simulink model "DemonstratorSimscape"  (R2020b)
settings: Solver=ode113  StartTime=0.0  StopTime=t_stop*0+20  FixedStep=1e-4
values from neighbouring files (symbols this model uses):
  brkD = 0    [main.m]
  brkI = 1e4    (= 10000)    [main.m]
  brkP = 1e5    (= 100000)    [main.m]
  d_drm = 0.5*d_drum    [main.m]
  d_shm = 0.4*d_sheave    [main.m]
  DeltaCable0 = 0    [main.m]
  Droop_scaling = 0    [main.m]
  eta_sh = 0.015    [main.m]
  filt_NUM = ones(1,200)*0.005    [main.m]
  g = 9.80665    [main.m]
  Iw = 0.5*(W.i + M.in*GB.r^2)    [main.m]
  Kp_mul = 0.3    [main.m]
  Lc0 = abs((T.ph-L.height-P.d-L.z0)*0.001)    [main.m]
  Ls1 = ((T.ph-0.5*W.pd)/1000)    [main.m]
  Ls2 = ((0.5*(T.s2+P.d)-2*P.d)/1000)    [main.m]
  M = 50e3    (= 50000)    [calcGrav.m]
  phi0_drm = -90    [main.m]
  phi0_shm = -90    [main.m]
  r_sheave = P.d*0.5    [main.m]
  s = tf('s')    [calcGrav.m]
  tau_brk = 0.001    [main.m]
  tau_em = 60e-3    (= 0.06)    [calcGrav.m]    (also in main.m)
  tau_m = tau_w/GB.r    [main.m]
  Tmax = 400e3    (= 400000)    [main.m]
  Tn_mul = 10    [main.m]
  x_drm = 0.7*r_drum    [main.m]
  x_shm = 0.7*r_sheave    [main.m]
  z0 = 0    [calcGrav.m]    (also in main.m = L.z0-P.d*0.5-P.d-P.d-L.height-T.h1-T.h2-32)
undefined symbols (not defined in the file or in its folder): C, CA, Controller_sampleTime, DiscIntNeverNeededParam, GB, L, P, Part, T, VFD_acceleration_model_factor, VFD_Adapt_factor_lower_p1458, VFD_Adapt_factor_upper_p1459, VFD_Curr_limit_var_p0641, VFD_Current_limit_p0640, VFD_Id_setp_total_r1624, VFD_Iq, VFD_Kp_n_basic_p1460, VFD_M, VFD_M_accel_T_smooth_p1517, VFD_M_lim_var_fixS_src_p1551, VFD_M_max_lower_p1521, VFD_M_max_lower_scal_p1525, VFD_M_max_up_mot_scal_p1524, VFD_M_max_upper_p1520, VFD_n_act_T_smooth_p1442, VFD_n_ctr_Kp_n_up_scal_p1461, VFD_n_ctr_Tn_n_up_sca_p1463, VFD_n_ctrl_adapt_Kp_lower_p1456, VFD_n_ctrl_adapt_Kp_upper_p1457, VFD_n_ctrl_Adpt_sig_Kp_p1455, VFD_n_ctrl_Kp_scal_p1466, VFD_n_ctrl_n_lower_p1464, VFD_n_ctrl_n_upper_p1465, VFD_n_ctrl_Tn_n_lower_p1462, VFD_n_limit_neg_p1086, VFD_n_limit_pos_p1083, VFD_n_limit_setp_p1063, VFD_n_max_p1082, VFD_n_set_filt_1_T_p1416, VFD_P_max_gen_p1531, VFD_P_max_mot_p1530, VFD_PU_I_outp_max_r0289, VFD_RFG_ramp_down_time_p1121, VFD_RFG_ramp_up_time_p1120, VFD_RFG_t_RD_scal_p1139, VFD_RFG_t_RU_scal_p1138, VSD, W, X, Y, Z
libraries: sm_lib x248, nesl_utility x128, simulink x49, pid_lib x4, cstblocks x2, simulink_extras x2
(part 4 of 10)

== system DemonstratorSimscape/Transmission System/Anchor and Load/CableFlex_Right ==
  disp [m] : Inport
  Inertia1 : sm_lib/Body Elements/Inertia  InertiaType=PointMass  Mass=0.00000001  MassUnits=kg  CenterOfMass=[0 0 0]  CenterOfMassUnits=m  MomentsOfInertia=[1 1 1]  MomentsOfInertiaUnits=kg*m^2  ProductsOfInertia=[0 0 0]  ProductsOfInertiaUnits=kg*m^2  GraphicType=None  MarkerShape=Inertia  MarkerSize=20  GraphicVisPropType=SimpleVisualProperties  GraphicDiffuseColor=[0.5 0.5 0.5]  GraphicSpecularColor=[0.5 0.5 0.5 1.0]  GraphicAmbientColor=[0.15 0.15 0.15 1.0]  GraphicEmissiveColor=[0.0 0.0 0.0 1.0]  GraphicShininess=75  GraphicOpacity=1.0
  Inertia2 : sm_lib/Body Elements/Inertia  InertiaType=PointMass  Mass=0.00000001  MassUnits=kg  CenterOfMass=[0 0 0]  CenterOfMassUnits=m  MomentsOfInertia=[1 1 1]  MomentsOfInertiaUnits=kg*m^2  ProductsOfInertia=[0 0 0]  ProductsOfInertiaUnits=kg*m^2  GraphicType=None  MarkerShape=Inertia  MarkerSize=20  GraphicVisPropType=SimpleVisualProperties  GraphicDiffuseColor=[0.5 0.5 0.5]  GraphicSpecularColor=[0.5 0.5 0.5 1.0]  GraphicAmbientColor=[0.15 0.15 0.15 1.0]  GraphicEmissiveColor=[0.0 0.0 0.0 1.0]  GraphicShininess=75  GraphicOpacity=1.0
  Prismatic Joint : sm_lib/Joints/Prismatic Joint  JointMode=Normal  SenseConstraintForce=off  SenseConstraintForceX=off  SenseConstraintForceY=off  SenseConstraintForceZ=off  SenseConstraintTorque=off  SenseConstraintTorqueX=off  SenseConstraintTorqueY=off  SenseConstraintTorqueZ=off  SenseTotalForce=off  SenseTotalForceX=off  SenseTotalForceY=off  SenseTotalForceZ=off  SenseTotalTorque=off  SenseTotalTorqueX=off  SenseTotalTorqueY=off  SenseTotalTorqueZ=off  CompositeWrenchDir=FollowerOnBase  CompositeWrenchFrame=BaseFrame  EquilibriumPosition=0  EquilibriumPositionUnits=m  SpringStiffness=0  SpringStiffnessUnits=N/m  DampingCoefficient=0  DampingCoefficientUnits=N/(m/s)  TorqueActuationMode=ComputedTorque  MotionActuationMode=InputMotion  SensePosition=off  SenseVelocity=off  SenseAcceleration=off  SenseTorqueForce=off  SenseLowerLimitTorqueForce=off  SenseUpperLimitTorqueForce=off  LowerLimitSpecify=off  LowerLimitBound=-1  LowerLimitBoundUnits=m  LowerLimitStiffness=1e6  LowerLimitStiffnessUnits=N/m  LowerLimitDamping=1e3  LowerLimitDampingUnits=N/(m/s)  LowerLimitTransitionRegionWidth=1e-4  LowerLimitTransitionRegionWidthUnits=m  UpperLimitSpecify=off  UpperLimitBound=1  UpperLimitBoundUnits=m  UpperLimitStiffness=1e6  UpperLimitStiffnessUnits=N/m  UpperLimitDamping=1e3  UpperLimitDampingUnits=N/(m/s)  UpperLimitTransitionRegionWidth=1e-4  UpperLimitTransitionRegionWidthUnits=m  PositionTargetSpecify=on  PositionTargetPriority=High  PositionTargetValue=DeltaCable0*0  PositionTargetValueUnits=mm  VelocityTargetSpecify=off  VelocityTargetPriority=High  VelocityTargetValue=0  VelocityTargetValueUnits=m/s
  Rigid Transform1 : sm_lib/Frames and Transforms/Rigid Transform  TranslationMethod=None  TranslationStandardOffset=0  TranslationLengthUnit=m  TranslationStandardAxis=+Z  TranslationCartesianOffset=[0 0 0]  TranslationROffset=0  TranslationROffsetUnits=m  TranslationZOffset=0  TranslationZOffsetUnits=m  TranslationThetaOffset=0  TranslationThetaOffsetUnits=deg  RotationMethod=StandardAxis  RotationAngleUnits=deg  RotationStandardAxis=+X  RotationAngle=-90  RotationArbitraryAxis=[0 0 1]  FollAlignAxisA=+X  BaseAlignAxisA=+Y  FollAlignAxisB=+Y  BaseAlignAxisB=+Z  RotationSequenceAxes=FollowerAxes  RotationSequence=XYX  RotationSequenceAngles=[0 0 0]  RotationSequenceAnglesUnits=deg  RotationMatrix=[1 0 0; 0 1 0; 0 0 1]
  Rigid Transform2 : sm_lib/Frames and Transforms/Rigid Transform  TranslationMethod=None  TranslationStandardOffset=0  TranslationLengthUnit=m  TranslationStandardAxis=+Z  TranslationCartesianOffset=[0 0 0]  TranslationROffset=0  TranslationROffsetUnits=m  TranslationZOffset=0  TranslationZOffsetUnits=m  TranslationThetaOffset=0  TranslationThetaOffsetUnits=deg  RotationMethod=StandardAxis  RotationAngleUnits=deg  RotationStandardAxis=+X  RotationAngle=90  RotationArbitraryAxis=[0 0 1]  FollAlignAxisA=+X  BaseAlignAxisA=+Y  FollAlignAxisB=+Y  BaseAlignAxisB=+Z  RotationSequenceAxes=FollowerAxes  RotationSequence=XYX  RotationSequenceAngles=[0 0 0]  RotationSequenceAnglesUnits=deg  RotationMatrix=[1 0 0; 0 1 0; 0 0 1]
  Simulink-PS Converter1 : nesl_utility/Simulink-PS Converter  PhysicalDomain=network_engine_domain  SubClassName=ps_input  LeftPortType=input  RightPortType=output  PseudoPeriodic=off  Frequencies=[]  NoiseDistribution=none  NoiseParameters=[]  Unit=m  AffineConversion=on  FilteringAndDerivatives=filter  SimscapeFilterOrder=2  InputFilterTimeConstant=0.001  UdotUserProvided=2
  F : PMIOPort  Side=Right
  B : PMIOPort  Port=2  Side=Left
  wires:
  disp [m]/1 -> Simulink-PS Converter1/1
  connections:
  B/RConn1 -- Rigid Transform2/LConn1
  Simulink-PS Converter1/RConn1 -- Prismatic Joint/LConn2
  Inertia2/RConn1 -- Prismatic Joint/LConn1 -- Rigid Transform1/LConn1
  Inertia1/RConn1 -- Prismatic Joint/RConn1 -- Rigid Transform2/RConn1
  F/RConn1 -- Rigid Transform1/RConn1

== system DemonstratorSimscape/Transmission System/Anchor and Load/CableRigid_Left ==
  F : PMIOPort  Side=Right
  B : PMIOPort  Port=2  Side=Left
  connections:
  B/RConn1 -- F/RConn1

== system DemonstratorSimscape/Transmission System/Anchor and Load/CableRigid_Right ==
  F : PMIOPort  Side=Right
  B : PMIOPort  Port=2  Side=Left
  connections:
  B/RConn1 -- F/RConn1

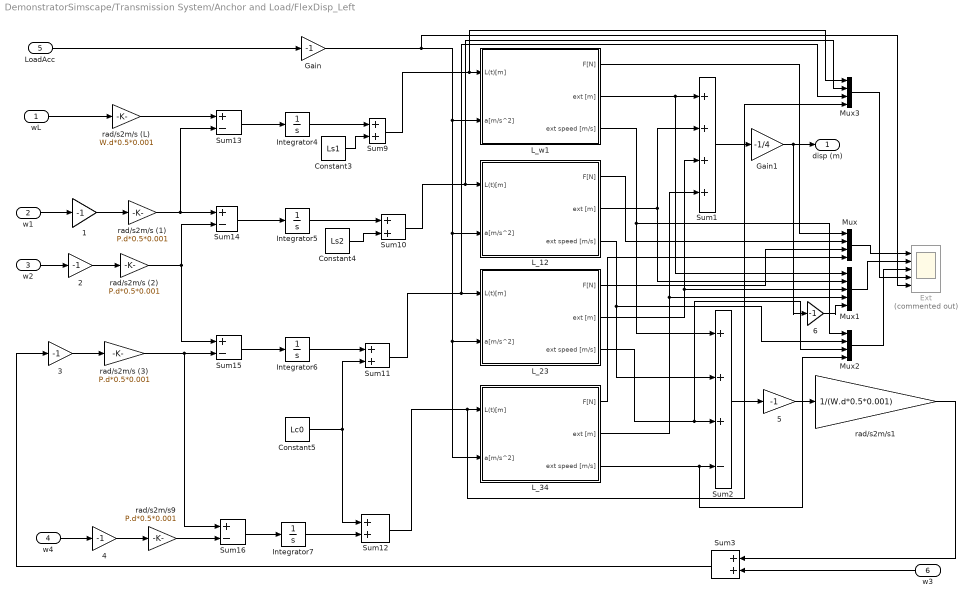
== system DemonstratorSimscape/Transmission System/Anchor and Load/FlexDisp_Left ==
  wL : Inport
  w1 : Inport  Port=2
  w2 : Inport  Port=3
  w4 : Inport  Port=4
  LoadAcc : Inport  Port=5
  w3 : Inport  Port=6
  {1..6} (6 alike) : Gain  Gain=-1
  Constant3 : Constant  Value=Ls1
  Constant4 : Constant  Value=Ls2
  Constant5 : Constant  Value=Lc0
  Ext : Scope  Commented=on  NumInputPorts=5
  Gain : Gain  Gain=-1
  Gain1 : Gain  Gain=-1/4
  Integrator{4..7} (4 alike) : Integrator
  L_12 : Subsystem
      settings: MinAlgLoopOccurrences=on
  L_23 : Subsystem
      settings: MinAlgLoopOccurrences=on
  L_34 : Subsystem
      settings: MinAlgLoopOccurrences=on
  L_w1 : Subsystem
      settings: MinAlgLoopOccurrences=on
  Mux : Mux
  Mux1 : Mux  Inputs=5
  Mux2 : Mux
  Mux3 : Mux
  Sum1 : Sum  Inputs=++++
  Sum{3,9..12} (5 alike) : Sum
  Sum{13..16} (4 alike) : Sum  Inputs=+-
  Sum2 : Sum  Inputs=+++-
  rad/s2m/s (1) : Gain  Gain=P.d*0.5*0.001
  rad/s2m/s (2) : Gain  Gain=P.d*0.5*0.001
  rad/s2m/s (3) : Gain  Gain=P.d*0.5*0.001
  rad/s2m/s (L) : Gain  Gain=W.d*0.5*0.001
  rad/s2m/s1 : Gain  Gain=1/(W.d*0.5*0.001)
  rad/s2m/s9 : Gain  Gain=P.d*0.5*0.001
  disp (m) : Outport
  wires:
  wL/1 -> rad/s2m/s (L)/1
  Integrator4/1 -> Sum9/1
  Sum15/1 -> Integrator6/1
  Sum9/1 -> Mux3/1, L_w1/1(L(t)[m])
  rad/s2m/s (1)/1 -> Sum14/1, Sum13/2
  LoadAcc/1 -> Gain/1
  Constant3/1 -> Sum9/2
  Sum12/1 -> Mux3/4, L_34/1(L(t)[m])
  Sum10/1 -> Mux3/2, L_12/1(L(t)[m])
  Integrator5/1 -> Sum10/1
  3/1 -> rad/s2m/s (3)/1
  2/1 -> rad/s2m/s (2)/1
  Sum13/1 -> Integrator4/1
  Constant5/1 -> Sum11/2, Sum12/1
  rad/s2m/s9/1 -> Sum16/2
  rad/s2m/s (L)/1 -> Sum13/1
  Integrator6/1 -> Sum11/1
  rad/s2m/s (3)/1 -> Sum15/2, Sum16/1
  w1/1 -> 1/1
  rad/s2m/s (2)/1 -> Sum14/2, Sum15/1
  4/1 -> rad/s2m/s9/1
  Constant4/1 -> Sum10/2
  Sum16/1 -> Integrator7/1
  w4/1 -> 4/1
  Sum14/1 -> Integrator5/1
  L_w1/2(ext [m]) -> Mux1/1, Sum1/1
  Sum11/1 -> Mux3/3, L_23/1(L(t)[m])
  1/1 -> rad/s2m/s (1)/1
  w2/1 -> 2/1
  Integrator7/1 -> Sum12/2
  Sum1/1 -> Gain1/1
  L_12/2(ext [m]) -> Sum1/2, Mux1/2
  L_23/2(ext [m]) -> Mux1/3, Sum1/3
  L_34/2(ext [m]) -> Mux1/4, Sum1/4
  Sum2/1 -> 5/1
  L_34/3(ext speed [m/s]) -> Mux2/4, Sum2/4
  L_23/3(ext speed [m/s]) -> Mux2/3, Sum2/3
  L_12/3(ext speed [m/s]) -> Mux2/2, Sum2/2
  L_w1/3(ext speed [m/s]) -> Mux2/1, Sum2/1
  5/1 -> rad/s2m/s1/1
  rad/s2m/s1/1 -> Sum3/1
  Sum3/1 -> 3/1
  Gain1/1 -> 6/1, disp (m)/1
  Gain/1 -> Ext/5, L_23/2(a[m/s^2]), L_34/2(a[m/s^2]), L_12/2(a[m/s^2]), L_w1/2(a[m/s^2])
  w3/1 -> Sum3/2
  Mux/1 -> Ext/1
  Mux1/1 -> Ext/2
  Mux2/1 -> Ext/3
  L_w1/1(F[N]) -> Mux/1
  L_12/1(F[N]) -> Mux/2
  L_23/1(F[N]) -> Mux/3
  L_34/1(F[N]) -> Mux/4
  6/1 -> Mux1/5
  Mux3/1 -> Ext/4

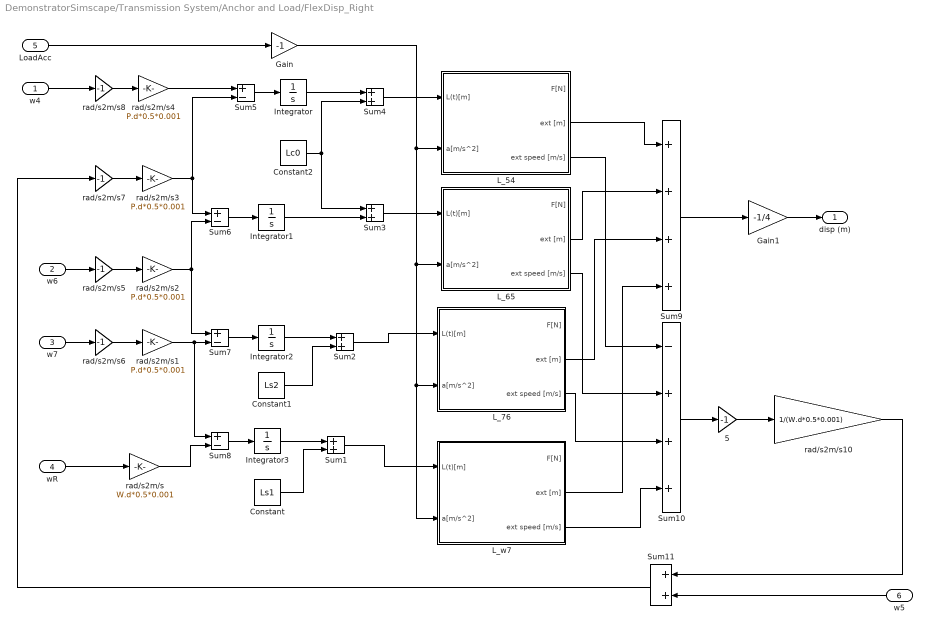
== system DemonstratorSimscape/Transmission System/Anchor and Load/FlexDisp_Right ==
  w4 : Inport
  w6 : Inport  Port=2
  w7 : Inport  Port=3
  wR : Inport  Port=4
  LoadAcc : Inport  Port=5
  w5 : Inport  Port=6
  5 : Gain  Gain=-1
  Constant : Constant  Value=Ls1
  Constant1 : Constant  Value=Ls2
  Constant2 : Constant  Value=Lc0
  Gain : Gain  Gain=-1
  Gain1 : Gain  Gain=-1/4
  Integrator{,1..3} (4 alike) : Integrator
  L_54 : Subsystem
      settings: MinAlgLoopOccurrences=on
  L_65 : Subsystem
      settings: MinAlgLoopOccurrences=on
  L_76 : Subsystem
      settings: MinAlgLoopOccurrences=on
  L_w7 : Subsystem
      settings: MinAlgLoopOccurrences=on
  Sum{1..4,11} (5 alike) : Sum
  Sum10 : Sum  Inputs=-+++
  Sum{5..8} (4 alike) : Sum  Inputs=+-
  Sum9 : Sum  Inputs=++++
  rad/s2m/s : Gain  Gain=W.d*0.5*0.001
  rad/s2m/s{1..4} (4 alike) : Gain  Gain=P.d*0.5*0.001
  rad/s2m/s10 : Gain  Gain=1/(W.d*0.5*0.001)
  rad/s2m/s{5..8} (4 alike) : Gain  Gain=-1
  disp (m) : Outport
  wires:
  Sum3/1 -> L_65/1(L(t)[m])
  w6/1 -> rad/s2m/s5/1
  LoadAcc/1 -> Gain/1
  Sum7/1 -> Integrator2/1
  Integrator/1 -> Sum4/1
  Sum4/1 -> L_54/1(L(t)[m])
  rad/s2m/s7/1 -> rad/s2m/s3/1
  rad/s2m/s3/1 -> Sum6/1, Sum5/2
  rad/s2m/s8/1 -> rad/s2m/s4/1
  w4/1 -> rad/s2m/s8/1
  rad/s2m/s6/1 -> rad/s2m/s1/1
  Constant2/1 -> Sum3/1, Sum4/2
  Sum8/1 -> Integrator3/1
  Sum2/1 -> L_76/1(L(t)[m])
  rad/s2m/s/1 -> Sum8/2
  Sum6/1 -> Integrator1/1
  Constant/1 -> Sum1/2
  rad/s2m/s5/1 -> rad/s2m/s2/1
  Sum5/1 -> Integrator/1
  Integrator2/1 -> Sum2/1
  rad/s2m/s2/1 -> Sum6/2, Sum7/1
  Constant1/1 -> Sum2/2
  Integrator1/1 -> Sum3/2
  Sum1/1 -> L_w7/1(L(t)[m])
  rad/s2m/s1/1 -> Sum7/2, Sum8/1
  w7/1 -> rad/s2m/s6/1
  Integrator3/1 -> Sum1/1
  rad/s2m/s4/1 -> Sum5/1
  wR/1 -> rad/s2m/s/1
  Gain/1 -> L_65/2(a[m/s^2]), L_76/2(a[m/s^2]), L_w7/2(a[m/s^2]), L_54/2(a[m/s^2])
  Sum9/1 -> Gain1/1
  L_54/2(ext [m]) -> Sum9/1
  L_65/2(ext [m]) -> Sum9/2
  L_76/2(ext [m]) -> Sum9/3
  L_w7/2(ext [m]) -> Sum9/4
  L_54/3(ext speed [m/s]) -> Sum10/1
  L_65/3(ext speed [m/s]) -> Sum10/2
  L_76/3(ext speed [m/s]) -> Sum10/3
  L_w7/3(ext speed [m/s]) -> Sum10/4
  rad/s2m/s10/1 -> Sum11/1
  Sum10/1 -> 5/1
  5/1 -> rad/s2m/s10/1
  Sum11/1 -> rad/s2m/s7/1
  w5/1 -> Sum11/2
  Gain1/1 -> disp (m)/1

== system DemonstratorSimscape/Transmission System/Anchor and Load/Load ==
  CableMass (kg) : Inport
  DOUBLE : Subsystem  Commented=on
  Load Sensors : Subsystem
  Pulley2 Rotation : sm_lib/Frames and Transforms/Rigid Transform  TranslationMethod=None  TranslationStandardOffset=0  TranslationLengthUnit=in  TranslationStandardAxis=+Z  TranslationCartesianOffset=[0 0 0]  TranslationROffset=0  TranslationROffsetUnits=m  TranslationZOffset=0  TranslationZOffsetUnits=m  TranslationThetaOffset=0  TranslationThetaOffsetUnits=deg  RotationMethod=StandardAxis  RotationAngleUnits=deg  RotationStandardAxis=+X  RotationAngle=-90  RotationArbitraryAxis=[0 0 1]  FollAlignAxisA=+Y  BaseAlignAxisA=+Z  FollAlignAxisB=+X  BaseAlignAxisB=+X  RotationSequenceAxes=FollowerAxes  RotationSequence=XYX  RotationSequenceAngles=[0 0 0]  RotationSequenceAnglesUnits=deg  RotationMatrix=[1 0 0; 0 1 0; 0 0 1]
  SINGLE : Subsystem
  F_Left : PMIOPort  Side=Left
  Centre : PMIOPort  Port=2  Side=Right
  F_Right : PMIOPort  Port=3  Side=Left
  LoadAcc (m/s^2) : Outport
  LoadPos (mm) : Outport  Port=2
  LoadVel (m/s) : Outport  Port=3
  wires:
  Load Sensors/2(LoadPos (mm)) -> LoadPos (mm)/1
  CableMass (kg)/1 -> DOUBLE/1(cable mass), SINGLE/1(cable mass)
  Load Sensors/1(LoadAcc (m/s^2)) -> LoadAcc (m/s^2)/1
  Load Sensors/3(LoadVel (m/s)) -> LoadVel (m/s)/1
  connections:
  DOUBLE/RConn2 -- F_Right/RConn1 -- SINGLE/RConn2
  SINGLE/LConn2 -- Load Sensors/RConn1 -- DOUBLE/LConn2
  SINGLE/LConn1 -- DOUBLE/LConn1 -- Pulley2 Rotation/RConn1
  DOUBLE/RConn1 -- SINGLE/RConn1 -- F_Left/RConn1
  Pulley2 Rotation/LConn1 -- Centre/RConn1

== system DemonstratorSimscape/Transmission System/Anchor and Load/Sheave_03 ==
  Bending loss : Subsystem  Commented=on
  Gain : Gain  Gain=-1
  Nm : nesl_utility/Simulink-PS Converter  PhysicalDomain=network_engine_domain  SubClassName=ps_input  LeftPortType=input  RightPortType=output  PseudoPeriodic=off  Frequencies=[]  NoiseDistribution=none  NoiseParameters=[]  Unit=1  AffineConversion=off  FilteringAndDerivatives=filter  SimscapeFilterOrder=2  InputFilterTimeConstant=tau_bending  UdotUserProvided=0
  PS>Sim1 : Subsystem
  Pulley 3 : sm_lib/Belts and Cables/Pulley  PitchRadius=P.d*0.5  PitchRadiusUnits=mm  InitialWrapAngleLowerBound=0.0  InitialWrapAngleLowerBoundUnits=deg  SenseWrapAngle=off  SensePulleyAngleA=off  SensePulleyAngleB=off  SenseFleetAngleA=off  SenseFleetAngleB=off
      settings: SourceProductBaseCode=MS
  Revolute Pulley3 : sm_lib/Joints/Revolute Joint  JointMode=Normal  SenseConstraintForce=on  SenseConstraintForceX=off  SenseConstraintForceY=off  SenseConstraintForceZ=off  SenseConstraintTorque=on  SenseConstraintTorqueX=off  SenseConstraintTorqueY=off  SenseConstraintTorqueZ=off  SenseTotalForce=on  SenseTotalForceX=off  SenseTotalForceY=off  SenseTotalForceZ=off  SenseTotalTorque=on  SenseTotalTorqueX=off  SenseTotalTorqueY=off  SenseTotalTorqueZ=off  CompositeWrenchDir=FollowerOnBase  CompositeWrenchFrame=BaseFrame  EquilibriumPosition=0  EquilibriumPositionUnits=deg  SpringStiffness=0  SpringStiffnessUnits=N*m/deg  DampingCoefficient=b_pulley  DampingCoefficientUnits=N*m/(deg/s)  TorqueActuationMode=InputTorque  MotionActuationMode=ComputedMotion  SensePosition=on  SenseVelocity=on  SenseAcceleration=on  SenseTorqueForce=on  SenseLowerLimitTorqueForce=off  SenseUpperLimitTorqueForce=off  LowerLimitSpecify=off  LowerLimitBound=-90  LowerLimitBoundUnits=deg  LowerLimitStiffness=1e4  LowerLimitStiffnessUnits=N*m/deg  LowerLimitDamping=10  LowerLimitDampingUnits=N*m/(deg/s)  LowerLimitTransitionRegionWidth=0.1  LowerLimitTransitionRegionWidthUnits=deg  UpperLimitSpecify=off  UpperLimitBound=90  UpperLimitBoundUnits=deg  UpperLimitStiffness=1e4  UpperLimitStiffnessUnits=N*m/deg  UpperLimitDamping=10  UpperLimitDampingUnits=N*m/(deg/s)  UpperLimitTransitionRegionWidth=0.1  UpperLimitTransitionRegionWidthUnits=deg  PositionTargetSpecify=off  PositionTargetPriority=High  PositionTargetValue=0  PositionTargetValueUnits=deg  VelocityTargetSpecify=off  VelocityTargetPriority=High  VelocityTargetValue=0  VelocityTargetValueUnits=deg/s
  ScopePulley3 : Scope  Commented=on  NumInputPorts=8
  Sheave3 : Subsystem
      mask Display: image('sm_cable_drive_right_angle_pulleyA_IMAGE.png');
  w0 (rad/s) : nesl_utility/PS-Simulink Converter  PhysicalDomain=network_engine_domain  SubClassName=ps_output  LeftPortType=input  RightPortType=output  PseudoPeriodic=off  Frequencies=[]  Unit=rad/s  AffineConversion=on
  WireA : PMIOPort  Side=Left
  ConnS3 : PMIOPort  Port=2  Side=Right
  WireB : PMIOPort  Port=3  Side=Left
  w (rad/s) : Outport
  tag scope: S3=global, w3=global
  wires:
  PS>Sim1/1(Out1) -> ScopePulley3/1
  PS>Sim1/2(Out2) -> ScopePulley3/2
  PS>Sim1/7(Out7) -> ScopePulley3/7
  PS>Sim1/3(Out3) -> ScopePulley3/3
  PS>Sim1/5(Out5) -> ScopePulley3/5
  PS>Sim1/4(Out4) -> ScopePulley3/4
  PS>Sim1/6(Out6) -> ScopePulley3/6
  PS>Sim1/8(Out8) -> ScopePulley3/8
  w0 (rad/s)/1 -> Gain/1, w (rad/s)/1
  [S2] -> Bending loss/1(Sin (kN))
  Bending loss/1(dT (Nm)) -> Nm/1
  Bending loss/2(Sout (kN)) -> [S3]
  Gain/1 -> [w3], Bending loss/2(w (deg/s))
  connections:
  Sheave3/LConn1 -- Revolute Pulley3/RConn1
  Revolute Pulley3/RConn9 -- PS>Sim1/LConn8
  Sheave3/RConn1 -- Pulley 3/LConn1
  WireA/RConn1 -- Pulley 3/RConn1
  Revolute Pulley3/RConn8 -- PS>Sim1/LConn7
  w0 (rad/s)/LConn1 -- Revolute Pulley3/RConn3 -- PS>Sim1/LConn2
  Revolute Pulley3/RConn4 -- PS>Sim1/LConn3
  Revolute Pulley3/RConn7 -- PS>Sim1/LConn6
  Revolute Pulley3/RConn5 -- PS>Sim1/LConn4
  Revolute Pulley3/RConn2 -- PS>Sim1/LConn1
  Revolute Pulley3/LConn1 -- ConnS3/RConn1
  Revolute Pulley3/RConn6 -- PS>Sim1/LConn5
  WireB/RConn1 -- Pulley 3/RConn2
  Nm/RConn1 -- Revolute Pulley3/LConn2

== system DemonstratorSimscape/Transmission System/Anchor and Load/Sheave_05 ==
  Bending loss : Subsystem  Commented=on
  Gain : Gain  Gain=-1
  Nm : nesl_utility/Simulink-PS Converter  PhysicalDomain=network_engine_domain  SubClassName=ps_input  LeftPortType=input  RightPortType=output  PseudoPeriodic=off  Frequencies=[]  NoiseDistribution=none  NoiseParameters=[]  Unit=1  AffineConversion=off  FilteringAndDerivatives=filter  SimscapeFilterOrder=2  InputFilterTimeConstant=tau_bending  UdotUserProvided=0
  PS>Sim2 : Subsystem
  Pulley 5 : sm_lib/Belts and Cables/Pulley  PitchRadius=P.d*0.5  PitchRadiusUnits=mm  InitialWrapAngleLowerBound=0.0  InitialWrapAngleLowerBoundUnits=deg  SenseWrapAngle=off  SensePulleyAngleA=off  SensePulleyAngleB=off  SenseFleetAngleA=off  SenseFleetAngleB=off
      settings: SourceProductBaseCode=MS
  Revolute Pulley5 : sm_lib/Joints/Revolute Joint  JointMode=Normal  SenseConstraintForce=on  SenseConstraintForceX=off  SenseConstraintForceY=off  SenseConstraintForceZ=off  SenseConstraintTorque=on  SenseConstraintTorqueX=off  SenseConstraintTorqueY=off  SenseConstraintTorqueZ=off  SenseTotalForce=on  SenseTotalForceX=off  SenseTotalForceY=off  SenseTotalForceZ=off  SenseTotalTorque=on  SenseTotalTorqueX=off  SenseTotalTorqueY=off  SenseTotalTorqueZ=off  CompositeWrenchDir=FollowerOnBase  CompositeWrenchFrame=BaseFrame  EquilibriumPosition=0  EquilibriumPositionUnits=deg  SpringStiffness=0  SpringStiffnessUnits=N*m/deg  DampingCoefficient=b_pulley  DampingCoefficientUnits=N*m/(deg/s)  TorqueActuationMode=InputTorque  MotionActuationMode=ComputedMotion  SensePosition=on  SenseVelocity=on  SenseAcceleration=on  SenseTorqueForce=on  SenseLowerLimitTorqueForce=off  SenseUpperLimitTorqueForce=off  LowerLimitSpecify=off  LowerLimitBound=-90  LowerLimitBoundUnits=deg  LowerLimitStiffness=1e4  LowerLimitStiffnessUnits=N*m/deg  LowerLimitDamping=10  LowerLimitDampingUnits=N*m/(deg/s)  LowerLimitTransitionRegionWidth=0.1  LowerLimitTransitionRegionWidthUnits=deg  UpperLimitSpecify=off  UpperLimitBound=90  UpperLimitBoundUnits=deg  UpperLimitStiffness=1e4  UpperLimitStiffnessUnits=N*m/deg  UpperLimitDamping=10  UpperLimitDampingUnits=N*m/(deg/s)  UpperLimitTransitionRegionWidth=0.1  UpperLimitTransitionRegionWidthUnits=deg  PositionTargetSpecify=off  PositionTargetPriority=High  PositionTargetValue=0  PositionTargetValueUnits=deg  VelocityTargetSpecify=off  VelocityTargetPriority=High  VelocityTargetValue=0  VelocityTargetValueUnits=deg/s
  ScopePulley5 : Scope  Commented=on  NumInputPorts=8
  Sheave5 : Subsystem
      mask Display: image('sm_cable_drive_right_angle_pulleyA_IMAGE.png');
  w (rad/s)1 : nesl_utility/PS-Simulink Converter  PhysicalDomain=network_engine_domain  SubClassName=ps_output  LeftPortType=input  RightPortType=output  PseudoPeriodic=off  Frequencies=[]  Unit=rad/s  AffineConversion=on
  ConnS5 : PMIOPort  Side=Right
  WireA : PMIOPort  Port=2  Side=Left
  WireB : PMIOPort  Port=3  Side=Left
  w (rad/s) : Outport
  tag scope: S4=global, w5=global
  wires:
  PS>Sim2/6(Out6) -> ScopePulley5/6
  PS>Sim2/3(Out3) -> ScopePulley5/3
  PS>Sim2/4(Out4) -> ScopePulley5/4
  PS>Sim2/7(Out7) -> ScopePulley5/7
  PS>Sim2/1(Out1) -> ScopePulley5/1
  PS>Sim2/5(Out5) -> ScopePulley5/5
  PS>Sim2/2(Out2) -> ScopePulley5/2
  PS>Sim2/8(Out8) -> ScopePulley5/8
  w (rad/s)1/1 -> Gain/1, w (rad/s)/1
  [S5] -> Bending loss/1(Sin (kN))
  Bending loss/1(dT (Nm)) -> Nm/1
  Bending loss/2(Sout (kN)) -> [S4]
  Gain/1 -> [w5], Bending loss/2(w (deg/s))
  connections:
  w (rad/s)1/LConn1 -- Revolute Pulley5/RConn3 -- PS>Sim2/LConn2
  WireB/RConn1 -- Pulley 5/RConn2
  Revolute Pulley5/RConn4 -- PS>Sim2/LConn3
  Revolute Pulley5/RConn6 -- PS>Sim2/LConn5
  Revolute Pulley5/RConn9 -- PS>Sim2/LConn8
  Revolute Pulley5/RConn7 -- PS>Sim2/LConn6
  Revolute Pulley5/RConn5 -- PS>Sim2/LConn4
  Revolute Pulley5/RConn8 -- PS>Sim2/LConn7
  Revolute Pulley5/RConn2 -- PS>Sim2/LConn1
  Sheave5/RConn1 -- Pulley 5/LConn1
  Sheave5/LConn1 -- Revolute Pulley5/RConn1
  Revolute Pulley5/LConn1 -- ConnS5/RConn1
  Pulley 5/RConn1 -- WireA/RConn1
  Nm/RConn1 -- Revolute Pulley5/LConn2

== system DemonstratorSimscape/Transmission System/Anchor and Load/cable mass ==
  "LoadPos [mm] " : Inport
  Add : Sum  Inputs=+-
  CableMass : Scope  Commented=on  NumInputPorts=2
  Constant : Constant  Value=P.up-W.pd*0.5
  Constant4 : Constant  Value=P.up
  Constant5 : Constant  Value=L.height
  Constant6 : Constant  Value=P.d
  Demux : Demux  Outputs=2
  Gain{,4,7,9} (4 alike) : Gain  Gain=CA.mpl
  Gain1 : Gain  Gain=2
  Gain10 : Gain  Gain=0.5
  Gain11 : Gain  Gain=0.5
  Gain12 : Gain  Gain=0.5
  Gain{2,5..6,8} (4 alike) : Gain  Gain=1/1000
  Gain3 : Gain  Gain=4
  Mux : Mux  Inputs=2
  Sum : Sum  Inputs=-+
  Sum1 : Sum  Inputs=+--
  Sum2 : Sum
  Sum3 : Sum
  net cable mass [kg] : Outport  VectorParamsAs1DForOutWhenUnconnected=off
  payout  [m] : Outport  Port=2  VectorParamsAs1DForOutWhenUnconnected=off
  cable mass [kg] : Outport  Port=3  VectorParamsAs1DForOutWhenUnconnected=off
  tag scope: LoadCableMass=global, WinchCableMass=global
  wires:
  Sum1/1 -> Gain3/1
  Constant5/1 -> Sum3/1
  Gain3/1 -> Add/1, Mux/2, Sum2/2, Sum/2
  Gain1/1 -> Add/2, Mux/1, Sum2/1, Sum/1
  Constant6/1 -> Sum3/2
  Constant4/1 -> Sum1/1
  Constant/1 -> Gain1/1
  Sum3/1 -> Sum1/2
  Sum/1 -> Gain5/1
  Gain/1 -> net cable mass [kg]/1
  Gain5/1 -> payout  [m]/1, Gain/1
  "LoadPos [mm] "/1 -> Sum1/3
  Mux/1 -> Gain6/1
  Gain6/1 -> Gain7/1
  Gain7/1 -> Gain10/1
  Sum2/1 -> Gain2/1
  Gain2/1 -> Gain4/1
  Gain4/1 -> cable mass [kg]/1
  Add/1 -> Gain8/1
  Gain8/1 -> Gain9/1
  Gain9/1 -> Gain11/1
  Gain10/1 -> Demux/1, CableMass/1
  Gain11/1 -> CableMass/2
  Gain12/1 -> [LoadCableMass]
  Demux/1 -> [WinchCableMass]
  Demux/2 -> Gain12/1

== system DemonstratorSimscape/Transmission System/Roof Pulley Set/ENDS ==
  Belt-Cable End : sm_lib/Belts and Cables/Belt-Cable End
      settings: SourceProductBaseCode=MS
  Belt-Cable End1 : sm_lib/Belts and Cables/Belt-Cable End
      settings: SourceProductBaseCode=MS
  Brick Solid : sm_lib/Body Elements/Brick Solid  GraphicAmbientColor=[0.15 0.15 0.15 1.0]  BasedOnType=Density  BrickDimensions=0.2*[1 1 1]  BrickDimensionUnits=m  CenterOfMass=[0 0 0]  CenterOfMassUnits=m  GraphicDiffuseColor=0.2*[1 1 1]  Density=0  DensityUnits=kg/m^3  DoExposeReferenceFrame=on  GraphicEmissiveColor=[0.0 0.0 0.0 1.0]  ExportEntireGeometry=off  SerializedFrames=<Frames/>  MarkerShape=Sphere  MarkerSize=10  GraphicType=FromGeometry  InertiaType=CalculateFromGeometry  Mass=1  MassUnits=kg  MomentsOfInertia=[1 1 1]  MomentsOfInertiaUnits=kg*m^2  GraphicOpacity=1.0  ProductsOfInertia=[0 0 0]  ProductsOfInertiaUnits=kg*m^2  GraphicShininess=75  GraphicSpecularColor=[0.5 0.5 0.5 1.0]  GraphicVisPropType=SimpleVisualProperties
  Brick Solid1 : sm_lib/Body Elements/Brick Solid  GraphicAmbientColor=[0.15 0.15 0.15 1.0]  BasedOnType=Density  BrickDimensions=0.2*[1 1 1]  BrickDimensionUnits=m  CenterOfMass=[0 0 0]  CenterOfMassUnits=m  GraphicDiffuseColor=0.2*[1 1 1]  Density=0  DensityUnits=kg/m^3  DoExposeReferenceFrame=on  GraphicEmissiveColor=[0.0 0.0 0.0 1.0]  ExportEntireGeometry=off  SerializedFrames=<Frames/>  MarkerShape=Sphere  MarkerSize=10  GraphicType=FromGeometry  InertiaType=CalculateFromGeometry  Mass=1  MassUnits=kg  MomentsOfInertia=[1 1 1]  MomentsOfInertiaUnits=kg*m^2  GraphicOpacity=1.0  ProductsOfInertia=[0 0 0]  ProductsOfInertiaUnits=kg*m^2  GraphicShininess=75  GraphicSpecularColor=[0.5 0.5 0.5 1.0]  GraphicVisPropType=SimpleVisualProperties
  Demux : Demux  Outputs=3
  Demux1 : Demux  Outputs=3
  Ends Tension : Scope  Commented=on
  Mux : Mux
  PS-Simulink Converter : nesl_utility/PS-Simulink Converter  PhysicalDomain=network_engine_domain  SubClassName=ps_output  LeftPortType=input  RightPortType=output  PseudoPeriodic=off  Frequencies=[]  Unit=kN  AffineConversion=off
  PS-Simulink Converter1 : nesl_utility/PS-Simulink Converter  PhysicalDomain=network_engine_domain  SubClassName=ps_output  LeftPortType=input  RightPortType=output  PseudoPeriodic=off  Frequencies=[]  Unit=kN  AffineConversion=off
  Rigid Transform1 : sm_lib/Frames and Transforms/Rigid Transform  TranslationMethod=Cartesian  TranslationStandardOffset=0  TranslationLengthUnit=mm  TranslationStandardAxis=+Z  TranslationCartesianOffset="[-P.Bd*0.5  0 0]"  TranslationROffset=0  TranslationROffsetUnits=m  TranslationZOffset=0  TranslationZOffsetUnits=m  TranslationThetaOffset=0  TranslationThetaOffsetUnits=deg  RotationMethod=None  RotationAngleUnits=deg  RotationStandardAxis=+Z  RotationAngle=0.0  RotationArbitraryAxis=[0 0 1]  FollAlignAxisA=+X  BaseAlignAxisA=+Y  FollAlignAxisB=+Y  BaseAlignAxisB=+Z  RotationSequenceAxes=FollowerAxes  RotationSequence=XYX  RotationSequenceAngles=[0 0 0]  RotationSequenceAnglesUnits=deg  RotationMatrix=[1 0 0; 0 1 0; 0 0 1]
  Rigid Transform3 : sm_lib/Frames and Transforms/Rigid Transform  TranslationMethod=Cartesian  TranslationStandardOffset=0  TranslationLengthUnit=mm  TranslationStandardAxis=+Z  TranslationCartesianOffset="[P.Bd*0.5  0 0]"  TranslationROffset=0  TranslationROffsetUnits=m  TranslationZOffset=0  TranslationZOffsetUnits=m  TranslationThetaOffset=0  TranslationThetaOffsetUnits=deg  RotationMethod=None  RotationAngleUnits=deg  RotationStandardAxis=+Z  RotationAngle=0.0  RotationArbitraryAxis=[0 0 1]  FollAlignAxisA=+X  BaseAlignAxisA=+Y  FollAlignAxisB=+Y  BaseAlignAxisB=+Z  RotationSequenceAxes=FollowerAxes  RotationSequence=XYX  RotationSequenceAngles=[0 0 0]  RotationSequenceAnglesUnits=deg  RotationMatrix=[1 0 0; 0 1 0; 0 0 1]
  Weld Joint : sm_lib/Joints/Weld Joint  JointMode=Normal  SenseConstraintForce=on  SenseConstraintForceX=off  SenseConstraintForceY=off  SenseConstraintForceZ=off  SenseConstraintTorque=off  SenseConstraintTorqueX=off  SenseConstraintTorqueY=off  SenseConstraintTorqueZ=off  SenseTotalForce=off  SenseTotalForceX=off  SenseTotalForceY=off  SenseTotalForceZ=off  SenseTotalTorque=off  SenseTotalTorqueX=off  SenseTotalTorqueY=off  SenseTotalTorqueZ=off  CompositeWrenchDir=BaseOnFollower  CompositeWrenchFrame=FollowerFrame
  Weld Joint1 : sm_lib/Joints/Weld Joint  JointMode=Normal  SenseConstraintForce=on  SenseConstraintForceX=off  SenseConstraintForceY=off  SenseConstraintForceZ=off  SenseConstraintTorque=off  SenseConstraintTorqueX=off  SenseConstraintTorqueY=off  SenseConstraintTorqueZ=off  SenseTotalForce=off  SenseTotalForceX=off  SenseTotalForceY=off  SenseTotalForceZ=off  SenseTotalTorque=off  SenseTotalTorqueX=off  SenseTotalTorqueY=off  SenseTotalTorqueZ=off  CompositeWrenchDir=BaseOnFollower  CompositeWrenchFrame=FollowerFrame
  ConnCentre : PMIOPort  Side=Left
  ConnEndL : PMIOPort  Port=2  Side=Right
  ConnEndR : PMIOPort  Port=3  Side=Right
  wires:
  PS-Simulink Converter/1 -> Demux/1
  PS-Simulink Converter1/1 -> Demux1/1
  Demux1/2 -> Mux/2
  Mux/1 -> Ends Tension/1
  Demux/2 -> Mux/1
  [S3] -> Mux/3
  [S4] -> Mux/4
  connections:
  ConnEndL/RConn1 -- Belt-Cable End1/RConn1
  Rigid Transform3/LConn1 -- Rigid Transform1/LConn1 -- ConnCentre/RConn1
  Weld Joint/RConn1 -- Belt-Cable End/LConn1
  Rigid Transform1/RConn1 -- Brick Solid1/RConn1 -- Weld Joint1/LConn1
  ConnEndR/RConn1 -- Belt-Cable End/RConn1
  Rigid Transform3/RConn1 -- Brick Solid/RConn1 -- Weld Joint/LConn1
  Weld Joint1/RConn1 -- Belt-Cable End1/LConn1
  Weld Joint/RConn2 -- PS-Simulink Converter/LConn1
  PS-Simulink Converter1/LConn1 -- Weld Joint1/RConn2

== system DemonstratorSimscape/Transmission System/Roof Pulley Set/Sheave_01 ==
  " " : sm_lib/Frames and Transforms/Rigid Transform  TranslationMethod=Cartesian  TranslationStandardOffset=0  TranslationLengthUnit=mm  TranslationStandardAxis=+Z  TranslationCartesianOffset=[0 -P.d*.25 -P.h]  TranslationROffset=0  TranslationROffsetUnits=m  TranslationZOffset=0  TranslationZOffsetUnits=m  TranslationThetaOffset=0  TranslationThetaOffsetUnits=deg  RotationMethod=ArbitraryAxis  RotationAngleUnits=deg  RotationStandardAxis=+Z  RotationAngle=90  RotationArbitraryAxis=[1 0 0]  FollAlignAxisA=+X  BaseAlignAxisA=+Y  FollAlignAxisB=+Y  BaseAlignAxisB=+Z  RotationSequenceAxes=FollowerAxes  RotationSequence=XYX  RotationSequenceAngles=[0 0 0]  RotationSequenceAnglesUnits=deg  RotationMatrix=[1 0 0; 0 1 0; 0 0 1]
  " 4" : sm_lib/Frames and Transforms/Rigid Transform  TranslationMethod=Cartesian  TranslationStandardOffset=0  TranslationLengthUnit=mm  TranslationStandardAxis=+Z  TranslationCartesianOffset=[0 -P.d*.25 P.h]  TranslationROffset=0  TranslationROffsetUnits=m  TranslationZOffset=0  TranslationZOffsetUnits=m  TranslationThetaOffset=0  TranslationThetaOffsetUnits=deg  RotationMethod=ArbitraryAxis  RotationAngleUnits=deg  RotationStandardAxis=+Z  RotationAngle=90  RotationArbitraryAxis=[1 0 0]  FollAlignAxisA=+X  BaseAlignAxisA=+Y  FollAlignAxisB=+Y  BaseAlignAxisB=+Z  RotationSequenceAxes=FollowerAxes  RotationSequence=XYX  RotationSequenceAngles=[0 0 0]  RotationSequenceAnglesUnits=deg  RotationMatrix=[1 0 0; 0 1 0; 0 0 1]
  Bending loss : Subsystem  Commented=on
  Gain : Gain
  Nm : nesl_utility/Simulink-PS Converter  PhysicalDomain=network_engine_domain  SubClassName=ps_input  LeftPortType=input  RightPortType=output  PseudoPeriodic=off  Frequencies=[]  NoiseDistribution=none  NoiseParameters=[]  Unit=1  AffineConversion=off  FilteringAndDerivatives=filter  SimscapeFilterOrder=2  InputFilterTimeConstant=tau_bending  UdotUserProvided=0
  PS>Sim1 : Subsystem
  Pulley 1 : sm_lib/Belts and Cables/Pulley  PitchRadius=P.d*0.5  PitchRadiusUnits=mm  InitialWrapAngleLowerBound=0.0  InitialWrapAngleLowerBoundUnits=deg  SenseWrapAngle=off  SensePulleyAngleA=off  SensePulleyAngleB=off  SenseFleetAngleA=off  SenseFleetAngleB=off
      settings: SourceProductBaseCode=MS
  Revolute Pulley1 : sm_lib/Joints/Revolute Joint  JointMode=Normal  SenseConstraintForce=on  SenseConstraintForceX=off  SenseConstraintForceY=off  SenseConstraintForceZ=off  SenseConstraintTorque=on  SenseConstraintTorqueX=off  SenseConstraintTorqueY=off  SenseConstraintTorqueZ=off  SenseTotalForce=on  SenseTotalForceX=off  SenseTotalForceY=off  SenseTotalForceZ=off  SenseTotalTorque=on  SenseTotalTorqueX=off  SenseTotalTorqueY=off  SenseTotalTorqueZ=off  CompositeWrenchDir=FollowerOnBase  CompositeWrenchFrame=BaseFrame  EquilibriumPosition=0  EquilibriumPositionUnits=deg  SpringStiffness=0  SpringStiffnessUnits=N*m/deg  DampingCoefficient=b_pulley  DampingCoefficientUnits=N*m/(deg/s)  TorqueActuationMode=InputTorque  MotionActuationMode=ComputedMotion  SensePosition=on  SenseVelocity=on  SenseAcceleration=on  SenseTorqueForce=on  SenseLowerLimitTorqueForce=off  SenseUpperLimitTorqueForce=off  LowerLimitSpecify=off  LowerLimitBound=-90  LowerLimitBoundUnits=deg  LowerLimitStiffness=1e4  LowerLimitStiffnessUnits=N*m/deg  LowerLimitDamping=10  LowerLimitDampingUnits=N*m/(deg/s)  LowerLimitTransitionRegionWidth=0.1  LowerLimitTransitionRegionWidthUnits=deg  UpperLimitSpecify=off  UpperLimitBound=90  UpperLimitBoundUnits=deg  UpperLimitStiffness=1e4  UpperLimitStiffnessUnits=N*m/deg  UpperLimitDamping=10  UpperLimitDampingUnits=N*m/(deg/s)  UpperLimitTransitionRegionWidth=0.1  UpperLimitTransitionRegionWidthUnits=deg  PositionTargetSpecify=off  PositionTargetPriority=High  PositionTargetValue=0  PositionTargetValueUnits=deg  VelocityTargetSpecify=off  VelocityTargetPriority=High  VelocityTargetValue=0  VelocityTargetValueUnits=deg/s
  ScopePulley1 : Scope  Commented=on  NumInputPorts=8
  Sheave1 : Subsystem
      mask Display: image('sm_cable_drive_right_angle_pulleyA_IMAGE.png');
  left face : sm_lib/Body Elements/Brick Solid  GraphicAmbientColor=[0.15 0.15 0.15 1.0]  BasedOnType=Density  BrickDimensions=[P.d P.h P.d*.5]  BrickDimensionUnits=mm  CenterOfMass=[0 0 0]  CenterOfMassUnits=m  GraphicDiffuseColor=[0.6 0.6 0.0]  Density=0  DensityUnits=g/cm^3  DoExposeReferenceFrame=on  GraphicEmissiveColor=[0.0 0.0 0.0 1.0]  ExportEntireGeometry=off  SerializedFrames=<Frames/>  MarkerShape=Sphere  MarkerSize=10  GraphicType=FromGeometry  InertiaType=CalculateFromGeometry  Mass=1  MassUnits=kg  MomentsOfInertia=[1 1 1]  MomentsOfInertiaUnits=kg*m^2  GraphicOpacity=c.opac  ProductsOfInertia=[0 0 0]  ProductsOfInertiaUnits=kg*m^2  GraphicShininess=75  GraphicSpecularColor=[0.5 0.5 0.5 1.0]  GraphicVisPropType=SimpleVisualProperties
  right face : sm_lib/Body Elements/Brick Solid  GraphicAmbientColor=[0.15 0.15 0.15 1.0]  BasedOnType=Density  BrickDimensions=[P.d P.h P.d*.5]  BrickDimensionUnits=mm  CenterOfMass=[0 0 0]  CenterOfMassUnits=m  GraphicDiffuseColor=[0.6 0.6 0.0]  Density=0  DensityUnits=g/cm^3  DoExposeReferenceFrame=on  GraphicEmissiveColor=[0.0 0.0 0.0 1.0]  ExportEntireGeometry=off  SerializedFrames=<Frames/>  MarkerShape=Sphere  MarkerSize=10  GraphicType=FromGeometry  InertiaType=CalculateFromGeometry  Mass=1  MassUnits=kg  MomentsOfInertia=[1 1 1]  MomentsOfInertiaUnits=kg*m^2  GraphicOpacity=1.0  ProductsOfInertia=[0 0 0]  ProductsOfInertiaUnits=kg*m^2  GraphicShininess=75  GraphicSpecularColor=[0.5 0.5 0.5 1.0]  GraphicVisPropType=SimpleVisualProperties
  w (rad/s)1 : nesl_utility/PS-Simulink Converter  PhysicalDomain=network_engine_domain  SubClassName=ps_output  LeftPortType=input  RightPortType=output  PseudoPeriodic=off  Frequencies=[]  Unit=rad/s  AffineConversion=off
  WireA : PMIOPort  Side=Right
  Conn1 : PMIOPort  Port=2  Side=Left
  WireB : PMIOPort  Port=3  Side=Right
  w (rad/s) : Outport
  tag scope: S1=global, w1=global
  wires:
  w (rad/s)1/1 -> [w1], Gain/1, w (rad/s)/1
  PS>Sim1/5(Out5) -> ScopePulley1/5
  PS>Sim1/8(Out8) -> ScopePulley1/8
  PS>Sim1/2(Out2) -> ScopePulley1/2
  PS>Sim1/1(Out1) -> ScopePulley1/1
  PS>Sim1/3(Out3) -> ScopePulley1/3
  PS>Sim1/7(Out7) -> ScopePulley1/7
  PS>Sim1/4(Out4) -> ScopePulley1/4
  PS>Sim1/6(Out6) -> ScopePulley1/6
  Bending loss/1(dT (Nm)) -> Nm/1
  Bending loss/2(Sout (kN)) -> [S1]
  [S0] -> Bending loss/1(Sin (kN))
  Gain/1 -> Bending loss/2(w (deg/s))
  connections:
  Pulley 1/RConn1 -- WireA/RConn1
  Sheave1/RConn1 -- Pulley 1/LConn1
  Pulley 1/RConn2 -- WireB/RConn1
  PS>Sim1/LConn2 -- Revolute Pulley1/RConn3 -- w (rad/s)1/LConn1
  " 4"/LConn1 -- " "/LConn1 -- Conn1/RConn1 -- Revolute Pulley1/LConn1
  Revolute Pulley1/RConn6 -- PS>Sim1/LConn5
  Revolute Pulley1/RConn2 -- PS>Sim1/LConn1
  Sheave1/LConn1 -- Revolute Pulley1/RConn1
  " "/RConn1 -- right face/RConn1
  Revolute Pulley1/RConn4 -- PS>Sim1/LConn3
  Revolute Pulley1/RConn9 -- PS>Sim1/LConn8
  Revolute Pulley1/RConn8 -- PS>Sim1/LConn7
  Revolute Pulley1/RConn5 -- PS>Sim1/LConn4
  Revolute Pulley1/RConn7 -- PS>Sim1/LConn6
  " 4"/RConn1 -- left face/RConn1
  Nm/RConn1 -- Revolute Pulley1/LConn2

== system DemonstratorSimscape/Transmission System/Roof Pulley Set/Sheave_02 ==
  " " : sm_lib/Frames and Transforms/Rigid Transform  TranslationMethod=Cartesian  TranslationStandardOffset=0  TranslationLengthUnit=mm  TranslationStandardAxis=+Z  TranslationCartesianOffset=[0 -P.d*.25 -P.h]  TranslationROffset=0  TranslationROffsetUnits=m  TranslationZOffset=0  TranslationZOffsetUnits=m  TranslationThetaOffset=0  TranslationThetaOffsetUnits=deg  RotationMethod=ArbitraryAxis  RotationAngleUnits=deg  RotationStandardAxis=+Z  RotationAngle=90  RotationArbitraryAxis=[1 0 0]  FollAlignAxisA=+X  BaseAlignAxisA=+Y  FollAlignAxisB=+Y  BaseAlignAxisB=+Z  RotationSequenceAxes=FollowerAxes  RotationSequence=XYX  RotationSequenceAngles=[0 0 0]  RotationSequenceAnglesUnits=deg  RotationMatrix=[1 0 0; 0 1 0; 0 0 1]
  " 4" : sm_lib/Frames and Transforms/Rigid Transform  TranslationMethod=Cartesian  TranslationStandardOffset=0  TranslationLengthUnit=mm  TranslationStandardAxis=+Z  TranslationCartesianOffset=[0 -P.d*.25 P.h]  TranslationROffset=0  TranslationROffsetUnits=m  TranslationZOffset=0  TranslationZOffsetUnits=m  TranslationThetaOffset=0  TranslationThetaOffsetUnits=deg  RotationMethod=ArbitraryAxis  RotationAngleUnits=deg  RotationStandardAxis=+Z  RotationAngle=90  RotationArbitraryAxis=[1 0 0]  FollAlignAxisA=+X  BaseAlignAxisA=+Y  FollAlignAxisB=+Y  BaseAlignAxisB=+Z  RotationSequenceAxes=FollowerAxes  RotationSequence=XYX  RotationSequenceAngles=[0 0 0]  RotationSequenceAnglesUnits=deg  RotationMatrix=[1 0 0; 0 1 0; 0 0 1]
  Bending loss : Subsystem  Commented=on
  Constant : Constant  Value=g*1000
  Demux : Demux  Outputs=3
  Divide : Product  Inputs=*/
  Gain : Gain
  Gain1 : Gain  Gain=-2
  Nm : nesl_utility/Simulink-PS Converter  PhysicalDomain=network_engine_domain  SubClassName=ps_input  LeftPortType=input  RightPortType=output  PseudoPeriodic=off  Frequencies=[]  NoiseDistribution=none  NoiseParameters=[]  Unit=1  AffineConversion=off  FilteringAndDerivatives=filter  SimscapeFilterOrder=2  InputFilterTimeConstant=tau_bending  UdotUserProvided=0
  PS>Sim1 : Subsystem
  Pulley 2 : sm_lib/Belts and Cables/Pulley  PitchRadius=P.d*0.5  PitchRadiusUnits=mm  InitialWrapAngleLowerBound=0.0  InitialWrapAngleLowerBoundUnits=deg  SenseWrapAngle=off  SensePulleyAngleA=off  SensePulleyAngleB=off  SenseFleetAngleA=off  SenseFleetAngleB=off
      settings: SourceProductBaseCode=MS
  Revolute Pulley2 : sm_lib/Joints/Revolute Joint  JointMode=Normal  SenseConstraintForce=on  SenseConstraintForceX=off  SenseConstraintForceY=off  SenseConstraintForceZ=off  SenseConstraintTorque=on  SenseConstraintTorqueX=off  SenseConstraintTorqueY=off  SenseConstraintTorqueZ=off  SenseTotalForce=on  SenseTotalForceX=off  SenseTotalForceY=off  SenseTotalForceZ=off  SenseTotalTorque=on  SenseTotalTorqueX=off  SenseTotalTorqueY=off  SenseTotalTorqueZ=off  CompositeWrenchDir=FollowerOnBase  CompositeWrenchFrame=BaseFrame  EquilibriumPosition=0  EquilibriumPositionUnits=deg  SpringStiffness=0  SpringStiffnessUnits=N*m/deg  DampingCoefficient=b_pulley  DampingCoefficientUnits=N*m/(deg/s)  TorqueActuationMode=InputTorque  MotionActuationMode=ComputedMotion  SensePosition=on  SenseVelocity=on  SenseAcceleration=on  SenseTorqueForce=on  SenseLowerLimitTorqueForce=off  SenseUpperLimitTorqueForce=off  LowerLimitSpecify=off  LowerLimitBound=-90  LowerLimitBoundUnits=deg  LowerLimitStiffness=1e4  LowerLimitStiffnessUnits=N*m/deg  LowerLimitDamping=10  LowerLimitDampingUnits=N*m/(deg/s)  LowerLimitTransitionRegionWidth=0.1  LowerLimitTransitionRegionWidthUnits=deg  UpperLimitSpecify=off  UpperLimitBound=90  UpperLimitBoundUnits=deg  UpperLimitStiffness=1e4  UpperLimitStiffnessUnits=N*m/deg  UpperLimitDamping=10  UpperLimitDampingUnits=N*m/(deg/s)  UpperLimitTransitionRegionWidth=0.1  UpperLimitTransitionRegionWidthUnits=deg  PositionTargetSpecify=off  PositionTargetPriority=High  PositionTargetValue=0  PositionTargetValueUnits=deg  VelocityTargetSpecify=off  VelocityTargetPriority=High  VelocityTargetValue=0  VelocityTargetValueUnits=deg/s
  ScopePulley2 : Scope  Commented=on  NumInputPorts=8
  Sheave2 : Subsystem
      mask Display: image('sm_cable_drive_right_angle_pulleyA_IMAGE.png');
  left face : sm_lib/Body Elements/Brick Solid  GraphicAmbientColor=[0.15 0.15 0.15 1.0]  BasedOnType=Density  BrickDimensions=[P.d P.h P.d*.5]  BrickDimensionUnits=mm  CenterOfMass=[0 0 0]  CenterOfMassUnits=m  GraphicDiffuseColor=[0.6 0.6 0.0]  Density=0  DensityUnits=g/cm^3  DoExposeReferenceFrame=on  GraphicEmissiveColor=[0.0 0.0 0.0 1.0]  ExportEntireGeometry=off  SerializedFrames=<Frames/>  MarkerShape=Sphere  MarkerSize=10  GraphicType=FromGeometry  InertiaType=CalculateFromGeometry  Mass=1  MassUnits=kg  MomentsOfInertia=[1 1 1]  MomentsOfInertiaUnits=kg*m^2  GraphicOpacity=c.opac  ProductsOfInertia=[0 0 0]  ProductsOfInertiaUnits=kg*m^2  GraphicShininess=75  GraphicSpecularColor=[0.5 0.5 0.5 1.0]  GraphicVisPropType=SimpleVisualProperties
  right face : sm_lib/Body Elements/Brick Solid  GraphicAmbientColor=[0.15 0.15 0.15 1.0]  BasedOnType=Density  BrickDimensions=[P.d P.h P.d*.5]  BrickDimensionUnits=mm  CenterOfMass=[0 0 0]  CenterOfMassUnits=m  GraphicDiffuseColor=[0.6 0.6 0.0]  Density=0  DensityUnits=g/cm^3  DoExposeReferenceFrame=on  GraphicEmissiveColor=[0.0 0.0 0.0 1.0]  ExportEntireGeometry=off  SerializedFrames=<Frames/>  MarkerShape=Sphere  MarkerSize=10  GraphicType=FromGeometry  InertiaType=CalculateFromGeometry  Mass=1  MassUnits=kg  MomentsOfInertia=[1 1 1]  MomentsOfInertiaUnits=kg*m^2  GraphicOpacity=1.0  ProductsOfInertia=[0 0 0]  ProductsOfInertiaUnits=kg*m^2  GraphicShininess=75  GraphicSpecularColor=[0.5 0.5 0.5 1.0]  GraphicVisPropType=SimpleVisualProperties
  w (rad/s)1 : nesl_utility/PS-Simulink Converter  PhysicalDomain=network_engine_domain  SubClassName=ps_output  LeftPortType=input  RightPortType=output  PseudoPeriodic=off  Frequencies=[]  Unit=rad/s  AffineConversion=off
  Conn1 : PMIOPort  Side=Left
  WireA : PMIOPort  Port=2  Side=Right
  WireB : PMIOPort  Port=3  Side=Right
  w (rad/s) : Outport
  tag scope: PinLoad_L_tonne=global, S2=global, w2=global
  wires:
  PS>Sim1/7(Out7) -> ScopePulley2/7
  w (rad/s)1/1 -> w (rad/s)/1, [w2], Gain/1
  PS>Sim1/2(Out2) -> ScopePulley2/2
  PS>Sim1/3(Out3) -> ScopePulley2/3
  PS>Sim1/8(Out8) -> ScopePulley2/8
  PS>Sim1/1(Out1) -> ScopePulley2/1
  PS>Sim1/5(Out5) -> Demux/1, ScopePulley2/5
  PS>Sim1/4(Out4) -> ScopePulley2/4
  PS>Sim1/6(Out6) -> ScopePulley2/6
  [S1] -> Bending loss/1(Sin (kN))
  Bending loss/2(Sout (kN)) -> [S2]
  Gain/1 -> Bending loss/2(w (deg/s))
  Bending loss/1(dT (Nm)) -> Nm/1
  Divide/1 -> [PinLoad_L_tonne]
  Gain1/1 -> Divide/1
  Constant/1 -> Divide/2
  Demux/2 -> Gain1/1
  connections:
  Sheave2/RConn1 -- Pulley 2/LConn1
  Pulley 2/RConn1 -- WireA/RConn1
  WireB/RConn1 -- Pulley 2/RConn2
  Revolute Pulley2/LConn1 -- Conn1/RConn1 -- " "/LConn1 -- " 4"/LConn1
  PS>Sim1/LConn2 -- w (rad/s)1/LConn1 -- Revolute Pulley2/RConn3
  Sheave2/LConn1 -- Revolute Pulley2/RConn1
  " "/RConn1 -- right face/RConn1
  Revolute Pulley2/RConn8 -- PS>Sim1/LConn7
  Revolute Pulley2/RConn6 -- PS>Sim1/LConn5
  " 4"/RConn1 -- left face/RConn1
  Revolute Pulley2/RConn2 -- PS>Sim1/LConn1
  Revolute Pulley2/RConn7 -- PS>Sim1/LConn6
  Revolute Pulley2/RConn5 -- PS>Sim1/LConn4
  Revolute Pulley2/RConn4 -- PS>Sim1/LConn3
  Revolute Pulley2/RConn9 -- PS>Sim1/LConn8
  Nm/RConn1 -- Revolute Pulley2/LConn2
